simulink model "simple"  (R2018a)
settings: Solver=FixedStepAuto  StartTime=0.0  StopTime=100  FixedStep=0.1  RelTol=1e-3
settings Model: Creator=clemw  LastModifiedBy=clemw

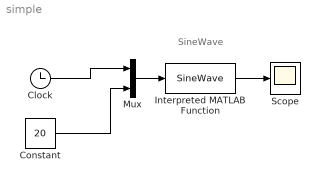
== system simple ==
  note: SineWave
  Clock : Clock
  Constant : Constant  Value=20
  Interpreted MATLAB Function : MATLABFcn  MATLABFcn=SineWave
  Mux : Mux  Inputs=2
  Scope : Scope
  wires:
  Interpreted MATLAB Function/1 -> Scope/1
  Mux/1 -> Interpreted MATLAB Function/1
  Clock/1 -> Mux/1
  Constant/1 -> Mux/2
